simulink model "StateSpaceLab2019b"  (R2019b)
settings: Solver=VariableStepAuto  StartTime=0.0  StopTime=4  RelTol=1e-3
settings Model: Creator=jakeabbott  LastModifiedBy=justinf

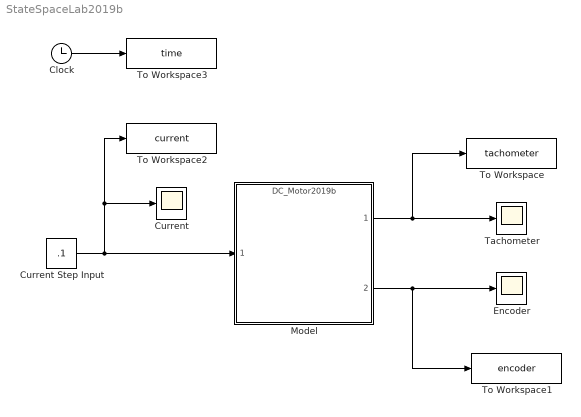
== system StateSpaceLab2019b ==
  Clock : Clock
  Current : Scope
  Current Step Input : Constant  Value=.1  SampleTime=0.001
  Encoder : Scope
  Model : ModelReference  ModelNameDialog=DC_Motor2019b.slxp  ModelReferenceVersion=1.20  CopyOfModelProtected=on
  Tachometer : Scope
  To Workspace : ToWorkspace  VariableName=tachometer  SampleTime=-1
  To Workspace1 : ToWorkspace  VariableName=encoder  SampleTime=-1
  To Workspace2 : ToWorkspace  VariableName=current  SampleTime=-1
  To Workspace3 : ToWorkspace  VariableName=time  SampleTime=-1
  wires:
  Current Step Input/1 -> Current/1, To Workspace2/1, Model/1
  Model/1 -> To Workspace/1, Tachometer/1
  Model/2 -> To Workspace1/1, Encoder/1
  Clock/1 -> To Workspace3/1
